simulink model "DDCU_wxt_v02_forA"  (R2014a)
settings: Solver=FixedStepDiscrete  StartTime=0.0  StopTime=50  FixedStep=0.0005  RelTol=1e-3
InitFcn:
  | Veh_Par_wxt
values from neighbouring files (symbols this model uses):
  ag_thr = 0.4*g    (= 3.924)    [Veh_Par_wxt.m]
  B = 2.25    [Veh_Par_wxt.m]
  bra_pre_em = 12    [Veh_Par_wxt.m]
  bra_pre_gz2 = 12/3    (= 4)    [Veh_Par_wxt.m]
  bra_pre_gz34 = 12/3    (= 4)    [Veh_Par_wxt.m]
  bra_pre_yd = 12/2    (= 6)    [Veh_Par_wxt.m]
  brakepre_dem_data = [0 1 2 3 4 5 6 7 8 9 10 11 12]    [Veh_Par_wxt.m]
  brakeTrq_dem_data = [0 218.198 436.396 654.594 872.792 1090.99 1309.188 1527.386 1745.584 1963.782 2181.98 2400.178 2618.376]    [Veh_Par_wxt.m]
  bratrq_max = 4*2618.376    (= 10473.504)    [Veh_Par_wxt.m]
  eff_tran = 0.75    [Veh_Par_wxt.m]
  G = Mass*g    (= 36297)    [Veh_Par_wxt.m]
  kd1 = 1    [Veh_Par_wxt.m]
  kd2 = 1    [Veh_Par_wxt.m]
  kd3 = 1    [Veh_Par_wxt.m]
  ki1 = 1    [Veh_Par_wxt.m]
  ki2 = 1    [Veh_Par_wxt.m]
  ki3 = 1    [Veh_Par_wxt.m]
  kp1 = 1    [Veh_Par_wxt.m]
  kp2 = 1    [Veh_Par_wxt.m]
  kp3 = 1    [Veh_Par_wxt.m]
  L = 3.12    [Veh_Par_wxt.m]
  Radius = 0.20    (= 0.2)    [Veh_Par_wxt.m]
  s_opt_yi_add = 0.05    [Veh_Par_wxt.m]
  s_opt_zhuan_add = 0.05    [Veh_Par_wxt.m]
  spd_map_mot = [0 100 200 300 360 400 500 600 700 800 900]*tras_ratio    [Veh_Par_wxt.m]
  speed_thr_park = 5/3.6/Radius*30/pi    (= 66.3145596216)    [Veh_Par_wxt.m]
  trq_map_mot = [1200 1200 1200 1200 1200 1080 864 720 617 540 480]/tras_ratio    [Veh_Par_wxt.m]
  v_thr1_b = 5    [Veh_Par_wxt.m]
  v_thr2_b = 20    [Veh_Par_wxt.m]
  v_thr_park = 5    [Veh_Par_wxt.m]
undefined symbols (not defined in the file or in its folder): DiscIntNeverNeededParam
libraries: simulink x201, ec5744lib x19
(part 9 of 9)

== matlab function DDCU_wxt_v02_forA/MainControl/mode_control/forward/forward/Brake/MATLAB Function5 ==
  data: bratrq_dem_lf input; bratrq_dem_lr input; bratrq_dem_rf input; bratrq_dem_rr input; flagyi_lf input; flagyi_lr input; bratrq_mot_lf output; flagyi_rf input; flagyi_rr input; bratrq_mot_lr output; bratrq_mot_rf output; bratrq_mot_rr output; bratrq_pid_lf input; bratrq_pid_lr input; bratrq_pid_rf input; bratrq_pid_rr input; brapre_out_l output; brapre_out_r output; gz_total input; v_act input; pwr_chg_bat input; trqlimL_dig_lf input; trqlimL_dig_lr input; trqlimL_dig_rf input; trqlimL_dig_rr input; speed_act_lf input; speed_act_lr input; speed_act_rf input; speed_act_rr input; v_thr1_b input; v_thr2_b input
function [bratrq_mot_lf,bratrq_mot_lr,bratrq_mot_rf,bratrq_mot_rr,brapre_out_l,brapre_out_r] = fcn(bratrq_dem_lf,bratrq_dem_lr,bratrq_dem_rf,bratrq_dem_rr,flagyi_lf,flagyi_lr,flagyi_rf,flagyi_rr,bratrq_pid_lf,bratrq_pid_lr,bratrq_pid_rf,bratrq_pid_rr,gz_total,v_act,pwr_chg_bat,trqlimL_dig_lf,trqlimL_dig_lr,trqlimL_dig_rf,trqlimL_dig_rr,speed_act_lf,speed_act_lr,speed_act_rf,speed_act_rr,v_thr1_b,v_thr2_b)
%#codegen pid模块在外面做，里面进行十六种情况的判断，先看一下效果，不能再修改。前轴单独控制，后轴低选控制
if flagyi_lf==0 && flagyi_lr==0 && flagyi_rf==0 && flagyi_rr==0 % 0电机滑移===============================================0电机滑移
    if gz_total==1  %电机有故障不进行制动能量回收，也不做ABS功能
        bratrq_mot_lf=0;
        bratrq_mot_lr=0;
        bratrq_mot_rf=0;
        bratrq_mot_rr=0;
        brapre_out_l=(bratrq_dem_lf+bratrq_dem_lr)/150;%除以150，对应Mpa
        brapre_out_r=(bratrq_dem_rf+bratrq_dem_rr)/150;
    else   %电机无故障，根据车速判断是否进行制动能量回收
        if   v_act<=v_thr1_b  %车速太小，机械制动
            bratrq_mot_lf=0;
            bratrq_mot_lr=0;
            bratrq_mot_rf=0;
            bratrq_mot_rr=0;
            brapre_out_l=(bratrq_dem_lf+bratrq_dem_lr)/150;%除以150，对应Mpa
            brapre_out_r=(bratrq_dem_rf+bratrq_dem_rr)/150;
        elseif v_act>v_thr1_b && v_act<=v_thr2_b %车速在5~20之间，复合制动
            bratrq_mot_lf1=bratrq_dem_lf*(v_act-v_thr1_b)/(v_thr2_b-v_thr1_b);
            bratrq_mot_lf2=9549*(pwr_chg_bat/4)/speed_act_lf;
            bratrq_mot_lf=min(trqlimL_dig_lf,min(bratrq_mot_lf1,bratrq_mot_lf2));
            
            bratrq_mot_lr1=bratrq_dem_lr*(v_act-v_thr1_b)/(v_thr2_b-v_thr1_b);
            bratrq_mot_lr2=9549*(pwr_chg_bat/4)/speed_act_lr;
            bratrq_mot_lr=min(trqlimL_dig_lr,min(bratrq_mot_lr1,bratrq_mot_lr2));
            
            bratrq_mot_rf1=bratrq_dem_rf*(v_act-v_thr1_b)/(v_thr2_b-v_thr1_b);
            bratrq_mot_rf2=9549*(pwr_chg_bat/4)/speed_act_rf;
            bratrq_mot_rf=min(trqlimL_dig_rf,min(bratrq_mot_rf1,bratrq_mot_rf2));
            
            bratrq_mot_rr1=bratrq_dem_rr*(v_act-v_thr1_b)/(v_thr2_b-v_thr1_b);
            bratrq_mot_rr2=9549*(pwr_chg_bat/4)/speed_act_rr;
            bratrq_mot_rr=min(trqlimL_dig_rr,min(bratrq_mot_rr1,bratrq_mot_rr2));
            
            brapre_out_l=((bratrq_dem_lf+bratrq_dem_lr)-(bratrq_mot_lf+bratrq_mot_lr))/150;
            brapre_out_r=((bratrq_dem_rf+bratrq_dem_rr)-(bratrq_mot_rf+bratrq_mot_rr))/150;
        else  %车速大于20，优先电制动
            bratrq_mot_lf1=bratrq_dem_lf;
            bratrq_mot_lf2=9549*(pwr_chg_bat/4)/speed_act_lf;
            bratrq_mot_lf=min(trqlimL_dig_lf,min(bratrq_mot_lf1,bratrq_mot_lf2));
            
            bratrq_mot_lr1=bratrq_dem_lr;
            bratrq_mot_lr2=9549*(pwr_chg_bat/4)/speed_act_lr;
            bratrq_mot_lr=min(trqlimL_dig_lr,min(bratrq_mot_lr1,bratrq_mot_lr2));
            
            bratrq_mot_rf1=bratrq_dem_rf;
            bratrq_mot_rf2=9549*(pwr_chg_bat/4)/speed_act_rf;
            bratrq_mot_rf=min(trqlimL_dig_rf,min(bratrq_mot_rf1,bratrq_mot_rf2));
            
            bratrq_mot_rr1=bratrq_dem_rr;
            bratrq_mot_rr2=9549*(pwr_chg_bat/4)/speed_act_rr;
            bratrq_mot_rr=min(trqlimL_dig_rr,min(bratrq_mot_rr1,bratrq_mot_rr2));
            
            brapre_out_l=((bratrq_dem_lf+bratrq_dem_lr)-(bratrq_mot_lf+bratrq_mot_lr))/150;
            brapre_out_r=((bratrq_dem_rf+bratrq_dem_rr)-(bratrq_mot_rf+bratrq_mot_rr))/150;
        end
    end
    
    
    
elseif flagyi_lf==1 && flagyi_lr==0 && flagyi_rf==0 && flagyi_rr==0 %左前轮滑移===================================================1电机滑移
    
    if gz_total==1  %电机有故障不进行制动能量回收，也不做ABS功能
        bratrq_mot_lf=0;
        bratrq_mot_lr=0;
        bratrq_mot_rf=0;
        bratrq_mot_rr=0;
        brapre_out_l=(bratrq_dem_lf+bratrq_dem_lr)/150;%除以150，对应Mpa
        brapre_out_r=(bratrq_dem_rf+bratrq_dem_rr)/150;
    else   %电机无故障，根据车速判断是否进行制动能量回收
        if   v_act<=v_thr1_b  %车速太小，机械制动
            bratrq_mot_lf=0;
            bratrq_mot_lr=0;
            bratrq_mot_rf=0;
            bratrq_mot_rr=0;
            brapre_out_l=(bratrq_dem_lf+bratrq_dem_lr)/150;%除以150，对应Mpa
            brapre_out_r=(bratrq_dem_rf+bratrq_dem_rr)/150;
        elseif v_act>v_thr1_b && v_act<=v_thr2_b %车速在5~20之间，复合制动
            bratrq_mot_lf1=bratrq_dem_lf*(v_act-v_thr1_b)/(v_thr2_b-v_thr1_b);
            bratrq_mot_lf2=9549*(pwr_chg_bat/4)/speed_act_lf;
            bratrq_mot_lf=min(trqlimL_dig_lf,min(bratrq_mot_lf1,bratrq_mot_lf2));
            
            bratrq_mot_lr1=bratrq_dem_lr*(v_act-v_thr1_b)/(v_thr2_b-v_thr1_b);
            bratrq_mot_lr2=9549*(pwr_chg_bat/4)/speed_act_lr;
            bratrq_mot_lr=min(trqlimL_dig_lr,min(bratrq_mot_lr1,bratrq_mot_lr2));
            
            bratrq_mot_rf1=bratrq_dem_rf*(v_act-v_thr1_b)/(v_thr2_b-v_thr1_b);
            bratrq_mot_rf2=9549*(pwr_chg_bat/4)/speed_act_rf;
            bratrq_mot_rf=min(trqlimL_dig_rf,min(bratrq_mot_rf1,bratrq_mot_rf2));
            
            bratrq_mot_rr1=bratrq_dem_rr*(v_act-v_thr1_b)/(v_thr2_b-v_thr1_b);
            bratrq_mot_rr2=9549*(pwr_chg_bat/4)/speed_act_rr;
            bratrq_mot_rr=min(trqlimL_dig_rr,min(bratrq_mot_rr1,bratrq_mot_rr2));
            
            brapre_out_l=((bratrq_dem_lf+bratrq_dem_lr)-(bratrq_mot_lf+bratrq_mot_lr))/150;
            brapre_out_r=((bratrq_dem_rf+bratrq_dem_rr)-(bratrq_mot_rf+bratrq_mot_rr))/150;
        else  %车速大于20，优先电制动,且进行ABS功能
            bratrq_mot_lf1=bratrq_dem_lf;
            bratrq_mot_lf2=9549*(pwr_chg_bat/4)/speed_act_lf;
            bratrq_mot_lf=min(trqlimL_dig_lf,min(bratrq_mot_lf1,bratrq_mot_lf2))+(bratrq_pid_lf-bratrq_dem_lf);
            
            bratrq_mot_lr1=bratrq_dem_lr;
            bratrq_mot_lr2=9549*(pwr_chg_bat/4)/speed_act_lr;
            bratrq_mot_lr=min(trqlimL_dig_lr,min(bratrq_mot_lr1,bratrq_mot_lr2));
            
            bratrq_mot_rf1=bratrq_dem_rf;
            bratrq_mot_rf2=9549*(pwr_chg_bat/4)/speed_act_rf;
            bratrq_mot_rf=min(trqlimL_dig_rf,min(bratrq_mot_rf1,bratrq_mot_rf2));
            
            bratrq_mot_rr1=bratrq_dem_rr;
            bratrq_mot_rr2=9549*(pwr_chg_bat/4)/speed_act_rr;
            bratrq_mot_rr=min(trqlimL_dig_rr,min(bratrq_mot_rr1,bratrq_mot_rr2));
            
            brapre_out_l=((bratrq_pid_lf+bratrq_dem_lr)-(bratrq_mot_lf+bratrq_mot_lr))/150;
            brapre_out_r=((bratrq_dem_rf+bratrq_dem_rr)-(bratrq_mot_rf+bratrq_mot_rr))/150;
        end
    end
    
    
elseif flagyi_lf==0 && flagyi_lr==1 && flagyi_rf==0 && flagyi_rr==0 %左后轮滑移,低选控制
    
    if gz_total==1  %电机有故障不进行制动能量回收，也不做ABS功能
        bratrq_mot_lf=0;
        bratrq_mot_lr=0;
        bratrq_mot_rf=0;
        bratrq_mot_rr=0;
        brapre_out_l=(bratrq_dem_lf+bratrq_dem_lr)/150;%除以150，对应Mpa
        brapre_out_r=(bratrq_dem_rf+bratrq_dem_rr)/150;
    else   %电机无故障，根据车速判断是否进行制动能量回收
        if   v_act<=v_thr1_b  %车速太小，机械制动
            bratrq_mot_lf=0;
            bratrq_mot_lr=0;
            bratrq_mot_rf=0;
            bratrq_mot_rr=0;
            brapre_out_l=(bratrq_dem_lf+bratrq_dem_lr)/150;%除以150，对应Mpa
            brapre_out_r=(bratrq_dem_rf+bratrq_dem_rr)/150;
        elseif v_act>v_thr1_b && v_act<=v_thr2_b %车速在5~20之间，复合制动
            bratrq_mot_lf1=bratrq_dem_lf*(v_act-v_thr1_b)/(v_thr2_b-v_thr1_b);
            bratrq_mot_lf2=9549*(pwr_chg_bat/4)/speed_act_lf;
            bratrq_mot_lf=min(trqlimL_dig_lf,min(bratrq_mot_lf1,bratrq_mot_lf2));
            
            bratrq_mot_lr1=bratrq_dem_lr*(v_act-v_thr1_b)/(v_thr2_b-v_thr1_b);
            bratrq_mot_lr2=9549*(pwr_chg_bat/4)/speed_act_lr;
            bratrq_mot_lr=min(trqlimL_dig_lr,min(bratrq_mot_lr1,bratrq_mot_lr2));
            
            bratrq_mot_rf1=bratrq_dem_rf*(v_act-v_thr1_b)/(v_thr2_b-v_thr1_b);
            bratrq_mot_rf2=9549*(pwr_chg_bat/4)/speed_act_rf;
            bratrq_mot_rf=min(trqlimL_dig_rf,min(bratrq_mot_rf1,bratrq_mot_rf2));
            
            bratrq_mot_rr1=bratrq_dem_rr*(v_act-v_thr1_b)/(v_thr2_b-v_thr1_b);
            bratrq_mot_rr2=9549*(pwr_chg_bat/4)/speed_act_rr;
            bratrq_mot_rr=min(trqlimL_dig_rr,min(bratrq_mot_rr1,bratrq_mot_rr2));
            
            brapre_out_l=((bratrq_dem_lf+bratrq_dem_lr)-(bratrq_mot_lf+bratrq_mot_lr))/150;
            brapre_out_r=((bratrq_dem_rf+bratrq_dem_rr)-(bratrq_mot_rf+bratrq_mot_rr))/150;
        else  %车速大于20，优先电制动,且进行ABS功能,左后降扭，右后同样得降扭啊。。。
            bratrq_mot_lf1=bratrq_dem_lf;
            bratrq_mot_lf2=9549*(pwr_chg_bat/4)/speed_act_lf;
            bratrq_mot_lf=min(trqlimL_dig_lf,min(bratrq_mot_lf1,bratrq_mot_lf2));
            
            bratrq_mot_lr1=bratrq_dem_lr;
            bratrq_mot_lr2=9549*(pwr_chg_bat/4)/speed_act_lr;
            bratrq_mot_lr=min(trqlimL_dig_lr,min(bratrq_mot_lr1,bratrq_mot_lr2))+(bratrq_pid_lr-bratrq_dem_lr);
            
            bratrq_mot_rf1=bratrq_dem_rf;
            bratrq_mot_rf2=9549*(pwr_chg_bat/4)/speed_act_rf;
            bratrq_mot_rf=min(trqlimL_dig_rf,min(bratrq_mot_rf1,bratrq_mot_rf2));
            
            bratrq_mot_rr1=bratrq_dem_rr;
            bratrq_mot_rr2=9549*(pwr_chg_bat/4)/speed_act_rr;
            bratrq_mot_rr=min(trqlimL_dig_rr,min(bratrq_mot_rr1,bratrq_mot_rr2))+(bratrq_pid_lr-bratrq_dem_lr);
            
            brapre_out_l=((bratrq_dem_lf+bratrq_pid_lr)-(bratrq_mot_lf+bratrq_mot_lr))/150;
            brapre_out_r=((bratrq_dem_rf+bratrq_dem_rr-(bratrq_pid_lr-bratrq_dem_lr))-(bratrq_mot_rf+bratrq_mot_rr))/150;
        end
    end
    
    
elseif flagyi_lf==0 && flagyi_lr==0 && flagyi_rf==1 && flagyi_rr==0 %右前轮滑移
    
    if gz_total==1  %电机有故障不进行制动能量回收，也不做ABS功能
        bratrq_mot_lf=0;
        bratrq_mot_lr=0;
        bratrq_mot_rf=0;
        bratrq_mot_rr=0;
        brapre_out_l=(bratrq_dem_lf+bratrq_dem_lr)/150;%除以150，对应Mpa
        brapre_out_r=(bratrq_dem_rf+bratrq_dem_rr)/150;
    else   %电机无故障，根据车速判断是否进行制动能量回收
        if   v_act<=v_thr1_b  %车速太小，机械制动
            bratrq_mot_lf=0;
            bratrq_mot_lr=0;
            bratrq_mot_rf=0;
            bratrq_mot_rr=0;
            brapre_out_l=(bratrq_dem_lf+bratrq_dem_lr)/150;%除以150，对应Mpa
            brapre_out_r=(bratrq_dem_rf+bratrq_dem_rr)/150;
        elseif v_act>v_thr1_b && v_act<=v_thr2_b %车速在5~20之间，复合制动
            bratrq_mot_lf1=bratrq_dem_lf*(v_act-v_thr1_b)/(v_thr2_b-v_thr1_b);
            bratrq_mot_lf2=9549*(pwr_chg_bat/4)/speed_act_lf;
            bratrq_mot_lf=min(trqlimL_dig_lf,min(bratrq_mot_lf1,bratrq_mot_lf2));
            
            bratrq_mot_lr1=bratrq_dem_lr*(v_act-v_thr1_b)/(v_thr2_b-v_thr1_b);
            bratrq_mot_lr2=9549*(pwr_chg_bat/4)/speed_act_lr;
            bratrq_mot_lr=min(trqlimL_dig_lr,min(bratrq_mot_lr1,bratrq_mot_lr2));
            
            bratrq_mot_rf1=bratrq_dem_rf*(v_act-v_thr1_b)/(v_thr2_b-v_thr1_b);
            bratrq_mot_rf2=9549*(pwr_chg_bat/4)/speed_act_rf;
            bratrq_mot_rf=min(trqlimL_dig_rf,min(bratrq_mot_rf1,bratrq_mot_rf2));
            
            bratrq_mot_rr1=bratrq_dem_rr*(v_act-v_thr1_b)/(v_thr2_b-v_thr1_b);
            bratrq_mot_rr2=9549*(pwr_chg_bat/4)/speed_act_rr;
            bratrq_mot_rr=min(trqlimL_dig_rr,min(bratrq_mot_rr1,bratrq_mot_rr2));
            
            brapre_out_l=((bratrq_dem_lf+bratrq_dem_lr)-(bratrq_mot_lf+bratrq_mot_lr))/150;
            brapre_out_r=((bratrq_dem_rf+bratrq_dem_rr)-(bratrq_mot_rf+bratrq_mot_rr))/150;
        else  %车速大于20，优先电制动,且进行ABS功能
            bratrq_mot_lf1=bratrq_dem_lf;
            bratrq_mot_lf2=9549*(pwr_chg_bat/4)/speed_act_lf;
            bratrq_mot_lf=min(trqlimL_dig_lf,min(bratrq_mot_lf1,bratrq_mot_lf2));
            
            bratrq_mot_lr1=bratrq_dem_lr;
            bratrq_mot_lr2=9549*(pwr_chg_bat/4)/speed_act_lr;
            bratrq_mot_lr=min(trqlimL_dig_lr,min(bratrq_mot_lr1,bratrq_mot_lr2));
            
            bratrq_mot_rf1=bratrq_dem_rf;
            bratrq_mot_rf2=9549*(pwr_chg_bat/4)/speed_act_rf;
            bratrq_mot_rf=min(trqlimL_dig_rf,min(bratrq_mot_rf1,bratrq_mot_rf2))+(bratrq_pid_rf-bratrq_dem_rf);
            
            bratrq_mot_rr1=bratrq_dem_rr;
            bratrq_mot_rr2=9549*(pwr_chg_bat/4)/speed_act_rr;
            bratrq_mot_rr=min(trqlimL_dig_rr,min(bratrq_mot_rr1,bratrq_mot_rr2));
            
            brapre_out_l=((bratrq_dem_lf+bratrq_dem_lr)-(bratrq_mot_lf+bratrq_mot_lr))/150;
            brapre_out_r=((bratrq_pid_rf+bratrq_dem_rr)-(bratrq_mot_rf+bratrq_mot_rr))/150;
        end
    end
    
    
elseif flagyi_lf==0 && flagyi_lr==0 && flagyi_rf==0 && flagyi_rr==1 %右后轮滑移
    
    if gz_total==1  %电机有故障不进行制动能量回收，也不做ABS功能
        bratrq_mot_lf=0;
        bratrq_mot_lr=0;
        bratrq_mot_rf=0;
        bratrq_mot_rr=0;
        brapre_out_l=(bratrq_dem_lf+bratrq_dem_lr)/150;%除以150，对应Mpa
        brapre_out_r=(bratrq_dem_rf+bratrq_dem_rr)/150;
    else   %电机无故障，根据车速判断是否进行制动能量回收
        if   v_act<=v_thr1_b  %车速太小，机械制动
            bratrq_mot_lf=0;
            bratrq_mot_lr=0;
            bratrq_mot_rf=0;
            bratrq_mot_rr=0;
            brapre_out_l=(bratrq_dem_lf+bratrq_dem_lr)/150;%除以150，对应Mpa
            brapre_out_r=(bratrq_dem_rf+bratrq_dem_rr)/150;
        elseif v_act>v_thr1_b && v_act<=v_thr2_b %车速在5~20之间，复合制动
            bratrq_mot_lf1=bratrq_dem_lf*(v_act-v_thr1_b)/(v_thr2_b-v_thr1_b);
            bratrq_mot_lf2=9549*(pwr_chg_bat/4)/speed_act_lf;
            bratrq_mot_lf=min(trqlimL_dig_lf,min(bratrq_mot_lf1,bratrq_mot_lf2));
            
            bratrq_mot_lr1=bratrq_dem_lr*(v_act-v_thr1_b)/(v_thr2_b-v_thr1_b);
            bratrq_mot_lr2=9549*(pwr_chg_bat/4)/speed_act_lr;
            bratrq_mot_lr=min(trqlimL_dig_lr,min(bratrq_mot_lr1,bratrq_mot_lr2));
            
            bratrq_mot_rf1=bratrq_dem_rf*(v_act-v_thr1_b)/(v_thr2_b-v_thr1_b);
            bratrq_mot_rf2=9549*(pwr_chg_bat/4)/speed_act_rf;
            bratrq_mot_rf=min(trqlimL_dig_rf,min(bratrq_mot_rf1,bratrq_mot_rf2));
            
            bratrq_mot_rr1=bratrq_dem_rr*(v_act-v_thr1_b)/(v_thr2_b-v_thr1_b);
            bratrq_mot_rr2=9549*(pwr_chg_bat/4)/speed_act_rr;
            bratrq_mot_rr=min(trqlimL_dig_rr,min(bratrq_mot_rr1,bratrq_mot_rr2));
            
            brapre_out_l=((bratrq_dem_lf+bratrq_dem_lr)-(bratrq_mot_lf+bratrq_mot_lr))/150;
            brapre_out_r=((bratrq_dem_rf+bratrq_dem_rr)-(bratrq_mot_rf+bratrq_mot_rr))/150;
        else  %车速大于20，优先电制动,且进行ABS功能,右后降扭，左后同样得降扭啊。。。
            
            bratrq_mot_rf1=bratrq_dem_rf;
            bratrq_mot_rf2=9549*(pwr_chg_bat/4)/speed_act_rf;
            bratrq_mot_rf=min(trqlimL_dig_rf,min(bratrq_mot_rf1,bratrq_mot_rf2));
            
            bratrq_mot_rr1=bratrq_dem_rr;
            bratrq_mot_rr2=9549*(pwr_chg_bat/4)/speed_act_rr;
            bratrq_mot_rr=min(trqlimL_dig_rr,min(bratrq_mot_rr1,bratrq_mot_rr2))+(bratrq_pid_rr-bratrq_dem_rr);
            
            bratrq_mot_lf1=bratrq_dem_lf;
            bratrq_mot_lf2=9549*(pwr_chg_bat/4)/speed_act_lf;
            bratrq_mot_lf=min(trqlimL_dig_lf,min(bratrq_mot_lf1,bratrq_mot_lf2));
            
            bratrq_mot_lr1=bratrq_dem_lr;
            bratrq_mot_lr2=9549*(pwr_chg_bat/4)/speed_act_lr;
            bratrq_mot_lr=min(trqlimL_dig_lr,min(bratrq_mot_lr1,bratrq_mot_lr2))+(bratrq_pid_rr-bratrq_dem_rr);
            
            
            
            brapre_out_l=((bratrq_dem_lf+bratrq_dem_lr-(bratrq_pid_rr-bratrq_dem_rr))-(bratrq_mot_lf+bratrq_mot_lr))/150;
            brapre_out_r=((bratrq_dem_rf+bratrq_pid_rr)-(bratrq_mot_rf+bratrq_mot_rr))/150;
        end
    end
    
    
elseif flagyi_lf==1 && flagyi_lr==1 && flagyi_rf==0 && flagyi_rr==0 %左侧两轮滑移=====================================================================2电机滑移
    
    if gz_total==1  %电机有故障不进行制动能量回收，也不做ABS功能
        bratrq_mot_lf=0;
        bratrq_mot_lr=0;
        bratrq_mot_rf=0;
        bratrq_mot_rr=0;
        brapre_out_l=(bratrq_dem_lf+bratrq_dem_lr)/150;%除以150，对应Mpa
        brapre_out_r=(bratrq_dem_rf+bratrq_dem_rr)/150;
    else   %电机无故障，根据车速判断是否进行制动能量回收
        if   v_act<=v_thr1_b  %车速太小，机械制动
            bratrq_mot_lf=0;
            bratrq_mot_lr=0;
            bratrq_mot_rf=0;
            bratrq_mot_rr=0;
            brapre_out_l=(bratrq_dem_lf+bratrq_dem_lr)/150;%除以150，对应Mpa
            brapre_out_r=(bratrq_dem_rf+bratrq_dem_rr)/150;
        elseif v_act>v_thr1_b && v_act<=v_thr2_b %车速在5~20之间，复合制动
            bratrq_mot_lf1=bratrq_dem_lf*(v_act-v_thr1_b)/(v_thr2_b-v_thr1_b);
            bratrq_mot_lf2=9549*(pwr_chg_bat/4)/speed_act_lf;
            bratrq_mot_lf=min(trqlimL_dig_lf,min(bratrq_mot_lf1,bratrq_mot_lf2));
            
            bratrq_mot_lr1=bratrq_dem_lr*(v_act-v_thr1_b)/(v_thr2_b-v_thr1_b);
            bratrq_mot_lr2=9549*(pwr_chg_bat/4)/speed_act_lr;
            bratrq_mot_lr=min(trqlimL_dig_lr,min(bratrq_mot_lr1,bratrq_mot_lr2));
            
            bratrq_mot_rf1=bratrq_dem_rf*(v_act-v_thr1_b)/(v_thr2_b-v_thr1_b);
            bratrq_mot_rf2=9549*(pwr_chg_bat/4)/speed_act_rf;
            bratrq_mot_rf=min(trqlimL_dig_rf,min(bratrq_mot_rf1,bratrq_mot_rf2));
            
            bratrq_mot_rr1=bratrq_dem_rr*(v_act-v_thr1_b)/(v_thr2_b-v_thr1_b);
            bratrq_mot_rr2=9549*(pwr_chg_bat/4)/speed_act_rr;
            bratrq_mot_rr=min(trqlimL_dig_rr,min(bratrq_mot_rr1,bratrq_mot_rr2));
            
            brapre_out_l=((bratrq_dem_lf+bratrq_dem_lr)-(bratrq_mot_lf+bratrq_mot_lr))/150;
            brapre_out_r=((bratrq_dem_rf+bratrq_dem_rr)-(bratrq_mot_rf+bratrq_mot_rr))/150;
        else  %车速大于20，优先电制动,且进行ABS功能
            bratrq_mot_lf1=bratrq_dem_lf;
            bratrq_mot_lf2=9549*(pwr_chg_bat/4)/speed_act_lf;
            bratrq_mot_lf=min(trqlimL_dig_lf,min(bratrq_mot_lf1,bratrq_mot_lf2))+(bratrq_pid_lf-bratrq_dem_lf);
            
            bratrq_mot_lr1=bratrq_dem_lr;
            bratrq_mot_lr2=9549*(pwr_chg_bat/4)/speed_act_lr;
            bratrq_mot_lr=min(trqlimL_dig_lr,min(bratrq_mot_lr1,bratrq_mot_lr2))+(bratrq_pid_lr-bratrq_dem_lr);
            
            bratrq_mot_rf1=bratrq_dem_rf;
            bratrq_mot_rf2=9549*(pwr_chg_bat/4)/speed_act_rf;
            bratrq_mot_rf=min(trqlimL_dig_rf,min(bratrq_mot_rf1,bratrq_mot_rf2));
            
            bratrq_mot_rr1=bratrq_dem_rr;
            bratrq_mot_rr2=9549*(pwr_chg_bat/4)/speed_act_rr;
            bratrq_mot_rr=min(trqlimL_dig_rr,min(bratrq_mot_rr1,bratrq_mot_rr2))+(bratrq_pid_lr-bratrq_dem_lr);
            
            brapre_out_l=((bratrq_pid_lf+bratrq_pid_lr)-(bratrq_mot_lf+bratrq_mot_lr))/150;
            brapre_out_r=((bratrq_dem_rf+bratrq_dem_rr-(bratrq_pid_lr-bratrq_dem_lr))-(bratrq_mot_rf+bratrq_mot_rr))/150;
        end
    end
    
    
elseif flagyi_lf==0 && flagyi_lr==0 && flagyi_rf==1 && flagyi_rr==1 %右侧两轮滑移
    
    if gz_total==1  %电机有故障不进行制动能量回收，也不做ABS功能
        bratrq_mot_lf=0;
        bratrq_mot_lr=0;
        bratrq_mot_rf=0;
        bratrq_mot_rr=0;
        brapre_out_l=(bratrq_dem_lf+bratrq_dem_lr)/150;%除以150，对应Mpa
        brapre_out_r=(bratrq_dem_rf+bratrq_dem_rr)/150;
    else   %电机无故障，根据车速判断是否进行制动能量回收
        if   v_act<=v_thr1_b  %车速太小，机械制动
            bratrq_mot_lf=0;
            bratrq_mot_lr=0;
            bratrq_mot_rf=0;
            bratrq_mot_rr=0;
            brapre_out_l=(bratrq_dem_lf+bratrq_dem_lr)/150;%除以150，对应Mpa
            brapre_out_r=(bratrq_dem_rf+bratrq_dem_rr)/150;
        elseif v_act>v_thr1_b && v_act<=v_thr2_b %车速在5~20之间，复合制动
            bratrq_mot_lf1=bratrq_dem_lf*(v_act-v_thr1_b)/(v_thr2_b-v_thr1_b);
            bratrq_mot_lf2=9549*(pwr_chg_bat/4)/speed_act_lf;
            bratrq_mot_lf=min(trqlimL_dig_lf,min(bratrq_mot_lf1,bratrq_mot_lf2));
            
            bratrq_mot_lr1=bratrq_dem_lr*(v_act-v_thr1_b)/(v_thr2_b-v_thr1_b);
            bratrq_mot_lr2=9549*(pwr_chg_bat/4)/speed_act_lr;
            bratrq_mot_lr=min(trqlimL_dig_lr,min(bratrq_mot_lr1,bratrq_mot_lr2));
            
            bratrq_mot_rf1=bratrq_dem_rf*(v_act-v_thr1_b)/(v_thr2_b-v_thr1_b);
            bratrq_mot_rf2=9549*(pwr_chg_bat/4)/speed_act_rf;
            bratrq_mot_rf=min(trqlimL_dig_rf,min(bratrq_mot_rf1,bratrq_mot_rf2));
            
            bratrq_mot_rr1=bratrq_dem_rr*(v_act-v_thr1_b)/(v_thr2_b-v_thr1_b);
            bratrq_mot_rr2=9549*(pwr_chg_bat/4)/speed_act_rr;
            bratrq_mot_rr=min(trqlimL_dig_rr,min(bratrq_mot_rr1,bratrq_mot_rr2));
            
            brapre_out_l=((bratrq_dem_lf+bratrq_dem_lr)-(bratrq_mot_lf+bratrq_mot_lr))/150;
            brapre_out_r=((bratrq_dem_rf+bratrq_dem_rr)-(bratrq_mot_rf+bratrq_mot_rr))/150;
        else  %车速大于20，优先电制动,且进行ABS功能
            bratrq_mot_rf1=bratrq_dem_rf;
            bratrq_mot_rf2=9549*(pwr_chg_bat/4)/speed_act_rf;
            bratrq_mot_rf=min(trqlimL_dig_rf,min(bratrq_mot_rf1,bratrq_mot_rf2))+(bratrq_pid_rf-bratrq_dem_rf);
            
            bratrq_mot_rr1=bratrq_dem_rr;
            bratrq_mot_rr2=9549*(pwr_chg_bat/4)/speed_act_rr;
            bratrq_mot_rr=min(trqlimL_dig_rr,min(bratrq_mot_rr1,bratrq_mot_rr2))+(bratrq_pid_rr-bratrq_dem_rr);
            
            bratrq_mot_lf1=bratrq_dem_lf;
            bratrq_mot_lf2=9549*(pwr_chg_bat/4)/speed_act_lf;
            bratrq_mot_lf=min(trqlimL_dig_lf,min(bratrq_mot_lf1,bratrq_mot_lf2));
            
            bratrq_mot_lr1=bratrq_dem_lr;
            bratrq_mot_lr2=9549*(pwr_chg_bat/4)/speed_act_lr;
            bratrq_mot_lr=min(trqlimL_dig_lr,min(bratrq_mot_lr1,bratrq_mot_lr2))+(bratrq_pid_rr-bratrq_dem_rr);
            
            
            
            brapre_out_l=((bratrq_pid_lf+bratrq_pid_lr-(bratrq_pid_rr-bratrq_dem_rr))-(bratrq_mot_lf+bratrq_mot_lr))/150;
            brapre_out_r=((bratrq_pid_rf+bratrq_pid_rr)-(bratrq_mot_rf+bratrq_mot_rr))/150;
        end
    end
    
    
elseif flagyi_lf==1 && flagyi_lr==0 && flagyi_rf==1 && flagyi_rr==0 %前轴滑移
    
    if gz_total==1  %电机有故障不进行制动能量回收，也不做ABS功能
        bratrq_mot_lf=0;
        bratrq_mot_lr=0;
        bratrq_mot_rf=0;
        bratrq_mot_rr=0;
        brapre_out_l=(bratrq_dem_lf+bratrq_dem_lr)/150;%除以150，对应Mpa
        brapre_out_r=(bratrq_dem_rf+bratrq_dem_rr)/150;
    else   %电机无故障，根据车速判断是否进行制动能量回收
        if   v_act<=v_thr1_b  %车速太小，机械制动
            bratrq_mot_lf=0;
            bratrq_mot_lr=0;
            bratrq_mot_rf=0;
            bratrq_mot_rr=0;
            brapre_out_l=(bratrq_dem_lf+bratrq_dem_lr)/150;%除以150，对应Mpa
            brapre_out_r=(bratrq_dem_rf+bratrq_dem_rr)/150;
        elseif v_act>v_thr1_b && v_act<=v_thr2_b %车速在5~20之间，复合制动
            bratrq_mot_lf1=bratrq_dem_lf*(v_act-v_thr1_b)/(v_thr2_b-v_thr1_b);
            bratrq_mot_lf2=9549*(pwr_chg_bat/4)/speed_act_lf;
            bratrq_mot_lf=min(trqlimL_dig_lf,min(bratrq_mot_lf1,bratrq_mot_lf2));
            
            bratrq_mot_lr1=bratrq_dem_lr*(v_act-v_thr1_b)/(v_thr2_b-v_thr1_b);
            bratrq_mot_lr2=9549*(pwr_chg_bat/4)/speed_act_lr;
            bratrq_mot_lr=min(trqlimL_dig_lr,min(bratrq_mot_lr1,bratrq_mot_lr2));
            
            bratrq_mot_rf1=bratrq_dem_rf*(v_act-v_thr1_b)/(v_thr2_b-v_thr1_b);
            bratrq_mot_rf2=9549*(pwr_chg_bat/4)/speed_act_rf;
            bratrq_mot_rf=min(trqlimL_dig_rf,min(bratrq_mot_rf1,bratrq_mot_rf2));
            
            bratrq_mot_rr1=bratrq_dem_rr*(v_act-v_thr1_b)/(v_thr2_b-v_thr1_b);
            bratrq_mot_rr2=9549*(pwr_chg_bat/4)/speed_act_rr;
            bratrq_mot_rr=min(trqlimL_dig_rr,min(bratrq_mot_rr1,bratrq_mot_rr2));
            
            brapre_out_l=((bratrq_dem_lf+bratrq_dem_lr)-(bratrq_mot_lf+bratrq_mot_lr))/150;
            brapre_out_r=((bratrq_dem_rf+bratrq_dem_rr)-(bratrq_mot_rf+bratrq_mot_rr))/150;
        else  %车速大于20，优先电制动,且进行ABS功能
            bratrq_mot_lf1=bratrq_dem_lf;
            bratrq_mot_lf2=9549*(pwr_chg_bat/4)/speed_act_lf;
            bratrq_mot_lf=min(trqlimL_dig_lf,min(bratrq_mot_lf1,bratrq_mot_lf2))+(bratrq_pid_lf-bratrq_dem_lf);
            
            bratrq_mot_lr1=bratrq_dem_lr;
            bratrq_mot_lr2=9549*(pwr_chg_bat/4)/speed_act_lr;
            bratrq_mot_lr=min(trqlimL_dig_lr,min(bratrq_mot_lr1,bratrq_mot_lr2));
            
            bratrq_mot_rf1=bratrq_dem_rf;
            bratrq_mot_rf2=9549*(pwr_chg_bat/4)/speed_act_rf;
            bratrq_mot_rf=min(trqlimL_dig_rf,min(bratrq_mot_rf1,bratrq_mot_rf2))+(bratrq_pid_rf-bratrq_dem_rf);
            
            bratrq_mot_rr1=bratrq_dem_rr;
            bratrq_mot_rr2=9549*(pwr_chg_bat/4)/speed_act_rr;
            bratrq_mot_rr=min(trqlimL_dig_rr,min(bratrq_mot_rr1,bratrq_mot_rr2));
            
            brapre_out_l=((bratrq_pid_lf+bratrq_dem_lr)-(bratrq_mot_lf+bratrq_mot_lr))/150;
            brapre_out_r=((bratrq_pid_rf+bratrq_dem_rr)-(bratrq_mot_rf+bratrq_mot_rr))/150;
        end
    end
    
    
elseif flagyi_lf==0 && flagyi_lr==1 && flagyi_rf==0 && flagyi_rr==1 %后轴滑移
    
    if gz_total==1  %电机有故障不进行制动能量回收，也不做ABS功能
        bratrq_mot_lf=0;
        bratrq_mot_lr=0;
        bratrq_mot_rf=0;
        bratrq_mot_rr=0;
        brapre_out_l=(bratrq_dem_lf+bratrq_dem_lr)/150;%除以150，对应Mpa
        brapre_out_r=(bratrq_dem_rf+bratrq_dem_rr)/150;
    else   %电机无故障，根据车速判断是否进行制动能量回收
        if   v_act<=v_thr1_b  %车速太小，机械制动
            bratrq_mot_lf=0;
            bratrq_mot_lr=0;
            bratrq_mot_rf=0;
            bratrq_mot_rr=0;
            brapre_out_l=(bratrq_dem_lf+bratrq_dem_lr)/150;%除以150，对应Mpa
            brapre_out_r=(bratrq_dem_rf+bratrq_dem_rr)/150;
        elseif v_act>v_thr1_b && v_act<=v_thr2_b %车速在5~20之间，复合制动
            bratrq_mot_lf1=bratrq_dem_lf*(v_act-v_thr1_b)/(v_thr2_b-v_thr1_b);
            bratrq_mot_lf2=9549*(pwr_chg_bat/4)/speed_act_lf;
            bratrq_mot_lf=min(trqlimL_dig_lf,min(bratrq_mot_lf1,bratrq_mot_lf2));
            
            bratrq_mot_lr1=bratrq_dem_lr*(v_act-v_thr1_b)/(v_thr2_b-v_thr1_b);
            bratrq_mot_lr2=9549*(pwr_chg_bat/4)/speed_act_lr;
            bratrq_mot_lr=min(trqlimL_dig_lr,min(bratrq_mot_lr1,bratrq_mot_lr2));
            
            bratrq_mot_rf1=bratrq_dem_rf*(v_act-v_thr1_b)/(v_thr2_b-v_thr1_b);
            bratrq_mot_rf2=9549*(pwr_chg_bat/4)/speed_act_rf;
            bratrq_mot_rf=min(trqlimL_dig_rf,min(bratrq_mot_rf1,bratrq_mot_rf2));
            
            bratrq_mot_rr1=bratrq_dem_rr*(v_act-v_thr1_b)/(v_thr2_b-v_thr1_b);
            bratrq_mot_rr2=9549*(pwr_chg_bat/4)/speed_act_rr;
            bratrq_mot_rr=min(trqlimL_dig_rr,min(bratrq_mot_rr1,bratrq_mot_rr2));
            
            brapre_out_l=((bratrq_dem_lf+bratrq_dem_lr)-(bratrq_mot_lf+bratrq_mot_lr))/150;
            brapre_out_r=((bratrq_dem_rf+bratrq_dem_rr)-(bratrq_mot_rf+bratrq_mot_rr))/150;
        else  %车速大于20，优先电制动,且进行ABS功能
            bratrq_mot_lf1=bratrq_dem_lf;
            bratrq_mot_lf2=9549*(pwr_chg_bat/4)/speed_act_lf;
            bratrq_mot_lf=min(trqlimL_dig_lf,min(bratrq_mot_lf1,bratrq_mot_lf2));
            
            bratrq_mot_rf1=bratrq_dem_rf;
            bratrq_mot_rf2=9549*(pwr_chg_bat/4)/speed_act_rf;
            bratrq_mot_rf=min(trqlimL_dig_rf,min(bratrq_mot_rf1,bratrq_mot_rf2));
            if (bratrq_pid_lr-bratrq_dem_lr)>(bratrq_pid_rr-bratrq_dem_rr)
                
                bratrq_mot_lr1=bratrq_dem_lr;
                bratrq_mot_lr2=9549*(pwr_chg_bat/4)/speed_act_lr;
                bratrq_mot_lr=min(trqlimL_dig_lr,min(bratrq_mot_lr1,bratrq_mot_lr2))+(bratrq_pid_rr-bratrq_dem_rr);
                
                
                
                bratrq_mot_rr1=bratrq_dem_rr;
                bratrq_mot_rr2=9549*(pwr_chg_bat/4)/speed_act_rr;
                bratrq_mot_rr=min(trqlimL_dig_rr,min(bratrq_mot_rr1,bratrq_mot_rr2))+(bratrq_pid_rr-bratrq_dem_rr);
                
                brapre_out_l=((bratrq_dem_lf+bratrq_dem_lr-(bratrq_pid_rr-bratrq_dem_rr))-(bratrq_mot_lf+bratrq_mot_lr))/150;
                brapre_out_r=((bratrq_dem_rf+bratrq_pid_rr)-(bratrq_mot_rf+bratrq_mot_rr))/150;
            else
                bratrq_mot_lr1=bratrq_dem_lr;
                bratrq_mot_lr2=9549*(pwr_chg_bat/4)/speed_act_lr;
                bratrq_mot_lr=min(trqlimL_dig_lr,min(bratrq_mot_lr1,bratrq_mot_lr2))+(bratrq_pid_lr-bratrq_dem_lr);
                
                
                
                bratrq_mot_rr1=bratrq_dem_rr;
                bratrq_mot_rr2=9549*(pwr_chg_bat/4)/speed_act_rr;
                bratrq_mot_rr=min(trqlimL_dig_rr,min(bratrq_mot_rr1,bratrq_mot_rr2))+(bratrq_pid_lr-bratrq_dem_lr);
                
                brapre_out_l=((bratrq_dem_lf+bratrq_pid_lr)-(bratrq_mot_lf+bratrq_mot_lr))/150;
                brapre_out_r=((bratrq_dem_rf+bratrq_dem_rr-(bratrq_pid_lr-bratrq_dem_lr))-(bratrq_mot_rf+bratrq_mot_rr))/150;
            end
        end
    end
    
    
elseif flagyi_lf==1 && flagyi_lr==0 && flagyi_rf==0 && flagyi_rr==1 %左前轮和右后轮滑移
    
    if gz_total==1  %电机有故障不进行制动能量回收，也不做ABS功能
        bratrq_mot_lf=0;
        bratrq_mot_lr=0;
        bratrq_mot_rf=0;
        bratrq_mot_rr=0;
        brapre_out_l=(bratrq_dem_lf+bratrq_dem_lr)/150;%除以150，对应Mpa
        brapre_out_r=(bratrq_dem_rf+bratrq_dem_rr)/150;
    else   %电机无故障，根据车速判断是否进行制动能量回收
        if   v_act<=v_thr1_b  %车速太小，机械制动
            bratrq_mot_lf=0;
            bratrq_mot_lr=0;
            bratrq_mot_rf=0;
            bratrq_mot_rr=0;
            brapre_out_l=(bratrq_dem_lf+bratrq_dem_lr)/150;%除以150，对应Mpa
            brapre_out_r=(bratrq_dem_rf+bratrq_dem_rr)/150;
        elseif v_act>v_thr1_b && v_act<=v_thr2_b %车速在5~20之间，复合制动
            bratrq_mot_lf1=bratrq_dem_lf*(v_act-v_thr1_b)/(v_thr2_b-v_thr1_b);
            bratrq_mot_lf2=9549*(pwr_chg_bat/4)/speed_act_lf;
            bratrq_mot_lf=min(trqlimL_dig_lf,min(bratrq_mot_lf1,bratrq_mot_lf2));
            
            bratrq_mot_lr1=bratrq_dem_lr*(v_act-v_thr1_b)/(v_thr2_b-v_thr1_b);
            bratrq_mot_lr2=9549*(pwr_chg_bat/4)/speed_act_lr;
            bratrq_mot_lr=min(trqlimL_dig_lr,min(bratrq_mot_lr1,bratrq_mot_lr2));
            
            bratrq_mot_rf1=bratrq_dem_rf*(v_act-v_thr1_b)/(v_thr2_b-v_thr1_b);
            bratrq_mot_rf2=9549*(pwr_chg_bat/4)/speed_act_rf;
            bratrq_mot_rf=min(trqlimL_dig_rf,min(bratrq_mot_rf1,bratrq_mot_rf2));
            
            bratrq_mot_rr1=bratrq_dem_rr*(v_act-v_thr1_b)/(v_thr2_b-v_thr1_b);
            bratrq_mot_rr2=9549*(pwr_chg_bat/4)/speed_act_rr;
            bratrq_mot_rr=min(trqlimL_dig_rr,min(bratrq_mot_rr1,bratrq_mot_rr2));
            
            brapre_out_l=((bratrq_dem_lf+bratrq_dem_lr)-(bratrq_mot_lf+bratrq_mot_lr))/150;
            brapre_out_r=((bratrq_dem_rf+bratrq_dem_rr)-(bratrq_mot_rf+bratrq_mot_rr))/150;
        else  %车速大于20，优先电制动,且进行ABS功能
            bratrq_mot_lf1=bratrq_dem_lf;
            bratrq_mot_lf2=9549*(pwr_chg_bat/4)/speed_act_lf;
            bratrq_mot_lf=min(trqlimL_dig_lf,min(bratrq_mot_lf1,bratrq_mot_lf2))+(bratrq_pid_lf-bratrq_dem_lf);
            
            bratrq_mot_rr1=bratrq_dem_rr;
            bratrq_mot_rr2=9549*(pwr_chg_bat/4)/speed_act_rr;
            bratrq_mot_rr=min(trqlimL_dig_rr,min(bratrq_mot_rr1,bratrq_mot_rr2))+(bratrq_pid_rr-bratrq_dem_rr);
            
            bratrq_mot_rf1=bratrq_dem_rf;
            bratrq_mot_rf2=9549*(pwr_chg_bat/4)/speed_act_rf;
            bratrq_mot_rf=min(trqlimL_dig_rf,min(bratrq_mot_rf1,bratrq_mot_rf2));
            
            bratrq_mot_lr1=bratrq_dem_lr;
            bratrq_mot_lr2=9549*(pwr_chg_bat/4)/speed_act_lr;
            bratrq_mot_lr=min(trqlimL_dig_lr,min(bratrq_mot_lr1,bratrq_mot_lr2))+(bratrq_pid_rr-bratrq_dem_rr);
            
            
            
            
            
            brapre_out_l=((bratrq_pid_lf+bratrq_dem_lr-(bratrq_pid_rr-bratrq_dem_rr))-(bratrq_mot_lf+bratrq_mot_lr))/150;
            brapre_out_r=((bratrq_dem_rf+bratrq_pid_rr)-(bratrq_mot_rf+bratrq_mot_rr))/150;
        end
    end
    
    
elseif flagyi_lf==0 && flagyi_lr==1 && flagyi_rf==1 && flagyi_rr==0 %左后轮和右前轮滑移
    
    if gz_total==1  %电机有故障不进行制动能量回收，也不做ABS功能
        bratrq_mot_lf=0;
        bratrq_mot_lr=0;
        bratrq_mot_rf=0;
        bratrq_mot_rr=0;
        brapre_out_l=(bratrq_dem_lf+bratrq_dem_lr)/150;%除以150，对应Mpa
        brapre_out_r=(bratrq_dem_rf+bratrq_dem_rr)/150;
    else   %电机无故障，根据车速判断是否进行制动能量回收
        if   v_act<=v_thr1_b  %车速太小，机械制动
            bratrq_mot_lf=0;
            bratrq_mot_lr=0;
            bratrq_mot_rf=0;
            bratrq_mot_rr=0;
            brapre_out_l=(bratrq_dem_lf+bratrq_dem_lr)/150;%除以150，对应Mpa
            brapre_out_r=(bratrq_dem_rf+bratrq_dem_rr)/150;
        elseif v_act>v_thr1_b && v_act<=v_thr2_b %车速在5~20之间，复合制动
            bratrq_mot_lf1=bratrq_dem_lf*(v_act-v_thr1_b)/(v_thr2_b-v_thr1_b);
            bratrq_mot_lf2=9549*(pwr_chg_bat/4)/speed_act_lf;
            bratrq_mot_lf=min(trqlimL_dig_lf,min(bratrq_mot_lf1,bratrq_mot_lf2));
            
            bratrq_mot_lr1=bratrq_dem_lr*(v_act-v_thr1_b)/(v_thr2_b-v_thr1_b);
            bratrq_mot_lr2=9549*(pwr_chg_bat/4)/speed_act_lr;
            bratrq_mot_lr=min(trqlimL_dig_lr,min(bratrq_mot_lr1,bratrq_mot_lr2));
            
            bratrq_mot_rf1=bratrq_dem_rf*(v_act-v_thr1_b)/(v_thr2_b-v_thr1_b);
            bratrq_mot_rf2=9549*(pwr_chg_bat/4)/speed_act_rf;
            bratrq_mot_rf=min(trqlimL_dig_rf,min(bratrq_mot_rf1,bratrq_mot_rf2));
            
            bratrq_mot_rr1=bratrq_dem_rr*(v_act-v_thr1_b)/(v_thr2_b-v_thr1_b);
            bratrq_mot_rr2=9549*(pwr_chg_bat/4)/speed_act_rr;
            bratrq_mot_rr=min(trqlimL_dig_rr,min(bratrq_mot_rr1,bratrq_mot_rr2));
            
            brapre_out_l=((bratrq_dem_lf+bratrq_dem_lr)-(bratrq_mot_lf+bratrq_mot_lr))/150;
            brapre_out_r=((bratrq_dem_rf+bratrq_dem_rr)-(bratrq_mot_rf+bratrq_mot_rr))/150;
        else  %车速大于20，优先电制动,且进行ABS功能
            
            bratrq_mot_rf1=bratrq_dem_rf;
            bratrq_mot_rf2=9549*(pwr_chg_bat/4)/speed_act_rf;
            bratrq_mot_rf=min(trqlimL_dig_rf,min(bratrq_mot_rf1,bratrq_mot_rf2))+(bratrq_pid_rf-bratrq_dem_rf);
            
            bratrq_mot_lr1=bratrq_dem_lr;
            bratrq_mot_lr2=9549*(pwr_chg_bat/4)/speed_act_lr;
            bratrq_mot_lr=min(trqlimL_dig_lr,min(bratrq_mot_lr1,bratrq_mot_lr2))+(bratrq_pid_lf-bratrq_dem_lf);
            
            bratrq_mot_lf1=bratrq_dem_lf;
            bratrq_mot_lf2=9549*(pwr_chg_bat/4)/speed_act_lf;
            bratrq_mot_lf=min(trqlimL_dig_lf,min(bratrq_mot_lf1,bratrq_mot_lf2));
            
            bratrq_mot_rr1=bratrq_dem_rr;
            bratrq_mot_rr2=9549*(pwr_chg_bat/4)/speed_act_rr;
            bratrq_mot_rr=min(trqlimL_dig_rr,min(bratrq_mot_rr1,bratrq_mot_rr2))+(bratrq_pid_lr-bratrq_dem_lr);
            
            brapre_out_l=((bratrq_dem_lf+bratrq_pid_lr)-(bratrq_mot_lf+bratrq_mot_lr))/150;
            brapre_out_r=((bratrq_pid_rf+bratrq_dem_rr-(bratrq_pid_lr-bratrq_dem_lr))-(bratrq_mot_rf+bratrq_mot_rr))/150;
        end
    end
    
    
elseif flagyi_lf==1 && flagyi_lr==1 && flagyi_rf==1 && flagyi_rr==0 %右后不滑移======================================================================3电机滑移
    
    if gz_total==1  %电机有故障不进行制动能量回收，也不做ABS功能
        bratrq_mot_lf=0;
        bratrq_mot_lr=0;
        bratrq_mot_rf=0;
        bratrq_mot_rr=0;
        brapre_out_l=(bratrq_dem_lf+bratrq_dem_lr)/150;%除以150，对应Mpa
        brapre_out_r=(bratrq_dem_rf+bratrq_dem_rr)/150;
    else   %电机无故障，根据车速判断是否进行制动能量回收
        if   v_act<=v_thr1_b  %车速太小，机械制动
            bratrq_mot_lf=0;
            bratrq_mot_lr=0;
            bratrq_mot_rf=0;
            bratrq_mot_rr=0;
            brapre_out_l=(bratrq_dem_lf+bratrq_dem_lr)/150;%除以150，对应Mpa
            brapre_out_r=(bratrq_dem_rf+bratrq_dem_rr)/150;
        elseif v_act>v_thr1_b && v_act<=v_thr2_b %车速在5~20之间，复合制动
            bratrq_mot_lf1=bratrq_dem_lf*(v_act-v_thr1_b)/(v_thr2_b-v_thr1_b);
            bratrq_mot_lf2=9549*(pwr_chg_bat/4)/speed_act_lf;
            bratrq_mot_lf=min(trqlimL_dig_lf,min(bratrq_mot_lf1,bratrq_mot_lf2));
            
            bratrq_mot_lr1=bratrq_dem_lr*(v_act-v_thr1_b)/(v_thr2_b-v_thr1_b);
            bratrq_mot_lr2=9549*(pwr_chg_bat/4)/speed_act_lr;
            bratrq_mot_lr=min(trqlimL_dig_lr,min(bratrq_mot_lr1,bratrq_mot_lr2));
            
            bratrq_mot_rf1=bratrq_dem_rf*(v_act-v_thr1_b)/(v_thr2_b-v_thr1_b);
            bratrq_mot_rf2=9549*(pwr_chg_bat/4)/speed_act_rf;
            bratrq_mot_rf=min(trqlimL_dig_rf,min(bratrq_mot_rf1,bratrq_mot_rf2));
            
            bratrq_mot_rr1=bratrq_dem_rr*(v_act-v_thr1_b)/(v_thr2_b-v_thr1_b);
            bratrq_mot_rr2=9549*(pwr_chg_bat/4)/speed_act_rr;
            bratrq_mot_rr=min(trqlimL_dig_rr,min(bratrq_mot_rr1,bratrq_mot_rr2));
            
            brapre_out_l=((bratrq_dem_lf+bratrq_dem_lr)-(bratrq_mot_lf+bratrq_mot_lr))/150;
            brapre_out_r=((bratrq_dem_rf+bratrq_dem_rr)-(bratrq_mot_rf+bratrq_mot_rr))/150;
        else  %车速大于20，优先电制动,且进行ABS功能
            bratrq_mot_lf1=bratrq_dem_lf;
            bratrq_mot_lf2=9549*(pwr_chg_bat/4)/speed_act_lf;
            bratrq_mot_lf=min(trqlimL_dig_lf,min(bratrq_mot_lf1,bratrq_mot_lf2))+(bratrq_pid_lf-bratrq_dem_lf);
            
            bratrq_mot_lr1=bratrq_dem_lr;
            bratrq_mot_lr2=9549*(pwr_chg_bat/4)/speed_act_lr;
            bratrq_mot_lr=min(trqlimL_dig_lr,min(bratrq_mot_lr1,bratrq_mot_lr2))+(bratrq_pid_lr-bratrq_dem_lr);
            
            bratrq_mot_rf1=bratrq_dem_rf;
            bratrq_mot_rf2=9549*(pwr_chg_bat/4)/speed_act_rf;
            bratrq_mot_rf=min(trqlimL_dig_rf,min(bratrq_mot_rf1,bratrq_mot_rf2))+(bratrq_pid_rf-bratrq_dem_rf);
            
            bratrq_mot_rr1=bratrq_dem_rr;
            bratrq_mot_rr2=9549*(pwr_chg_bat/4)/speed_act_rr;
            bratrq_mot_rr=min(trqlimL_dig_rr,min(bratrq_mot_rr1,bratrq_mot_rr2))+(bratrq_pid_lr-bratrq_dem_lr);
            
            brapre_out_l=((bratrq_pid_lf+bratrq_pid_lr)-(bratrq_mot_lf+bratrq_mot_lr))/150;
            brapre_out_r=((bratrq_pid_rf+bratrq_dem_rr-(bratrq_pid_lr-bratrq_dem_lr))-(bratrq_mot_rf+bratrq_mot_rr))/150;
        end
    end
    
    
elseif flagyi_lf==1 && flagyi_lr==1 && flagyi_rf==0 && flagyi_rr==1 %右前不滑移
    
    if gz_total==1  %电机有故障不进行制动能量回收，也不做ABS功能
        bratrq_mot_lf=0;
        bratrq_mot_lr=0;
        bratrq_mot_rf=0;
        bratrq_mot_rr=0;
        brapre_out_l=(bratrq_dem_lf+bratrq_dem_lr)/150;%除以150，对应Mpa
        brapre_out_r=(bratrq_dem_rf+bratrq_dem_rr)/150;
    else   %电机无故障，根据车速判断是否进行制动能量回收
        if   v_act<=v_thr1_b  %车速太小，机械制动
            bratrq_mot_lf=0;
            bratrq_mot_lr=0;
            bratrq_mot_rf=0;
            bratrq_mot_rr=0;
            brapre_out_l=(bratrq_dem_lf+bratrq_dem_lr)/150;%除以150，对应Mpa
            brapre_out_r=(bratrq_dem_rf+bratrq_dem_rr)/150;
        elseif v_act>v_thr1_b && v_act<=v_thr2_b %车速在5~20之间，复合制动
            bratrq_mot_lf1=bratrq_dem_lf*(v_act-v_thr1_b)/(v_thr2_b-v_thr1_b);
            bratrq_mot_lf2=9549*(pwr_chg_bat/4)/speed_act_lf;
            bratrq_mot_lf=min(trqlimL_dig_lf,min(bratrq_mot_lf1,bratrq_mot_lf2));
            
            bratrq_mot_lr1=bratrq_dem_lr*(v_act-v_thr1_b)/(v_thr2_b-v_thr1_b);
            bratrq_mot_lr2=9549*(pwr_chg_bat/4)/speed_act_lr;
            bratrq_mot_lr=min(trqlimL_dig_lr,min(bratrq_mot_lr1,bratrq_mot_lr2));
            
            bratrq_mot_rf1=bratrq_dem_rf*(v_act-v_thr1_b)/(v_thr2_b-v_thr1_b);
            bratrq_mot_rf2=9549*(pwr_chg_bat/4)/speed_act_rf;
            bratrq_mot_rf=min(trqlimL_dig_rf,min(bratrq_mot_rf1,bratrq_mot_rf2));
            
            bratrq_mot_rr1=bratrq_dem_rr*(v_act-v_thr1_b)/(v_thr2_b-v_thr1_b);
            bratrq_mot_rr2=9549*(pwr_chg_bat/4)/speed_act_rr;
            bratrq_mot_rr=min(trqlimL_dig_rr,min(bratrq_mot_rr1,bratrq_mot_rr2));
            
            brapre_out_l=((bratrq_dem_lf+bratrq_dem_lr)-(bratrq_mot_lf+bratrq_mot_lr))/150;
            brapre_out_r=((bratrq_dem_rf+bratrq_dem_rr)-(bratrq_mot_rf+bratrq_mot_rr))/150;
        else  %车速大于20，优先电制动,且进行ABS功能
            bratrq_mot_lf1=bratrq_dem_lf;
            bratrq_mot_lf2=9549*(pwr_chg_bat/4)/speed_act_lf;
            bratrq_mot_lf=min(trqlimL_dig_lf,min(bratrq_mot_lf1,bratrq_mot_lf2))+(bratrq_pid_lf-bratrq_dem_lf);
            
            bratrq_mot_rf1=bratrq_dem_rf;
            bratrq_mot_rf2=9549*(pwr_chg_bat/4)/speed_act_rf;
            bratrq_mot_rf=min(trqlimL_dig_rf,min(bratrq_mot_rf1,bratrq_mot_rf2));
            
            if (bratrq_pid_lr-bratrq_dem_lr)>(bratrq_pid_rr-bratrq_dem_rr)
                
                bratrq_mot_lr1=bratrq_dem_lr;
                bratrq_mot_lr2=9549*(pwr_chg_bat/4)/speed_act_lr;
                bratrq_mot_lr=min(trqlimL_dig_lr,min(bratrq_mot_lr1,bratrq_mot_lr2))+(bratrq_pid_rr-bratrq_dem_rr);
                
                
                
                bratrq_mot_rr1=bratrq_dem_rr;
                bratrq_mot_rr2=9549*(pwr_chg_bat/4)/speed_act_rr;
                bratrq_mot_rr=min(trqlimL_dig_rr,min(bratrq_mot_rr1,bratrq_mot_rr2))+(bratrq_pid_rr-bratrq_dem_rr);
                
                brapre_out_l=((bratrq_pid_lf+bratrq_dem_lr-(bratrq_pid_rr-bratrq_dem_rr))-(bratrq_mot_lf+bratrq_mot_lr))/150;
                brapre_out_r=((bratrq_dem_rf+bratrq_pid_rr)-(bratrq_mot_rf+bratrq_mot_rr))/150;
                
            else
                bratrq_mot_lr1=bratrq_dem_lr;
                bratrq_mot_lr2=9549*(pwr_chg_bat/4)/speed_act_lr;
                bratrq_mot_lr=min(trqlimL_dig_lr,min(bratrq_mot_lr1,bratrq_mot_lr2))+(bratrq_pid_lr-bratrq_dem_lr);
                
                
                
                bratrq_mot_rr1=bratrq_dem_rr;
                bratrq_mot_rr2=9549*(pwr_chg_bat/4)/speed_act_rr;
                bratrq_mot_rr=min(trqlimL_dig_rr,min(bratrq_mot_rr1,bratrq_mot_rr2))+(bratrq_pid_lr-bratrq_dem_lr);
                
                brapre_out_l=((bratrq_pid_lf+bratrq_pid_lr)-(bratrq_mot_lf+bratrq_mot_lr))/150;
                brapre_out_r=((bratrq_dem_rf+bratrq_dem_rr-(bratrq_pid_lr-bratrq_dem_lr))-(bratrq_mot_rf+bratrq_mot_rr))/150;
            end
        end
    end
    
    
elseif flagyi_lf==1 && flagyi_lr==0 && flagyi_rf==1 && flagyi_rr==1 %左后不滑移
    
    if gz_total==1  %电机有故障不进行制动能量回收，也不做ABS功能
        bratrq_mot_lf=0;
        bratrq_mot_lr=0;
        bratrq_mot_rf=0;
        bratrq_mot_rr=0;
        brapre_out_l=(bratrq_dem_lf+bratrq_dem_lr)/150;%除以150，对应Mpa
        brapre_out_r=(bratrq_dem_rf+bratrq_dem_rr)/150;
    else   %电机无故障，根据车速判断是否进行制动能量回收
        if   v_act<=v_thr1_b  %车速太小，机械制动
            bratrq_mot_lf=0;
            bratrq_mot_lr=0;
            bratrq_mot_rf=0;
            bratrq_mot_rr=0;
            brapre_out_l=(bratrq_dem_lf+bratrq_dem_lr)/150;%除以150，对应Mpa
            brapre_out_r=(bratrq_dem_rf+bratrq_dem_rr)/150;
        elseif v_act>v_thr1_b && v_act<=v_thr2_b %车速在5~20之间，复合制动
            bratrq_mot_lf1=bratrq_dem_lf*(v_act-v_thr1_b)/(v_thr2_b-v_thr1_b);
            bratrq_mot_lf2=9549*(pwr_chg_bat/4)/speed_act_lf;
            bratrq_mot_lf=min(trqlimL_dig_lf,min(bratrq_mot_lf1,bratrq_mot_lf2));
            
            bratrq_mot_lr1=bratrq_dem_lr*(v_act-v_thr1_b)/(v_thr2_b-v_thr1_b);
            bratrq_mot_lr2=9549*(pwr_chg_bat/4)/speed_act_lr;
            bratrq_mot_lr=min(trqlimL_dig_lr,min(bratrq_mot_lr1,bratrq_mot_lr2));
            
            bratrq_mot_rf1=bratrq_dem_rf*(v_act-v_thr1_b)/(v_thr2_b-v_thr1_b);
            bratrq_mot_rf2=9549*(pwr_chg_bat/4)/speed_act_rf;
            bratrq_mot_rf=min(trqlimL_dig_rf,min(bratrq_mot_rf1,bratrq_mot_rf2));
            
            bratrq_mot_rr1=bratrq_dem_rr*(v_act-v_thr1_b)/(v_thr2_b-v_thr1_b);
            bratrq_mot_rr2=9549*(pwr_chg_bat/4)/speed_act_rr;
            bratrq_mot_rr=min(trqlimL_dig_rr,min(bratrq_mot_rr1,bratrq_mot_rr2));
            
            brapre_out_l=((bratrq_dem_lf+bratrq_dem_lr)-(bratrq_mot_lf+bratrq_mot_lr))/150;
            brapre_out_r=((bratrq_dem_rf+bratrq_dem_rr)-(bratrq_mot_rf+bratrq_mot_rr))/150;
        else  %车速大于20，优先电制动,且进行ABS功能
            bratrq_mot_lf1=bratrq_dem_lf;
            bratrq_mot_lf2=9549*(pwr_chg_bat/4)/speed_act_lf;
            bratrq_mot_lf=min(trqlimL_dig_lf,min(bratrq_mot_lf1,bratrq_mot_lf2))+(bratrq_pid_lf-bratrq_dem_lf);
            
            bratrq_mot_rf1=bratrq_dem_rf;
            bratrq_mot_rf2=9549*(pwr_chg_bat/4)/speed_act_rf;
            bratrq_mot_rf=min(trqlimL_dig_rf,min(bratrq_mot_rf1,bratrq_mot_rf2))+(bratrq_pid_rf-bratrq_dem_rf);
            
            
            bratrq_mot_rr1=bratrq_dem_rr;
            bratrq_mot_rr2=9549*(pwr_chg_bat/4)/speed_act_rr;
            bratrq_mot_rr=min(trqlimL_dig_rr,min(bratrq_mot_rr1,bratrq_mot_rr2))+(bratrq_pid_rr-bratrq_dem_rr);
            
            bratrq_mot_lr1=bratrq_dem_lr;
            bratrq_mot_lr2=9549*(pwr_chg_bat/4)/speed_act_lr;
            bratrq_mot_lr=min(trqlimL_dig_lr,min(bratrq_mot_lr1,bratrq_mot_lr2))+(bratrq_pid_rr-bratrq_dem_rr);
            
            
            
            
            brapre_out_l=((bratrq_pid_lf+bratrq_dem_lr-(bratrq_pid_rr-bratrq_dem_rr))-(bratrq_mot_lf+bratrq_mot_lr))/150;
            brapre_out_r=((bratrq_pid_rf+bratrq_pid_rr)-(bratrq_mot_rf+bratrq_mot_rr))/150;
        end
    end
    
    
elseif flagyi_lf==0 && flagyi_lr==1 && flagyi_rf==1 && flagyi_rr==1 %左前不滑移
    
    if gz_total==1  %电机有故障不进行制动能量回收，也不做ABS功能
        bratrq_mot_lf=0;
        bratrq_mot_lr=0;
        bratrq_mot_rf=0;
        bratrq_mot_rr=0;
        brapre_out_l=(bratrq_dem_lf+bratrq_dem_lr)/150;%除以150，对应Mpa
        brapre_out_r=(bratrq_dem_rf+bratrq_dem_rr)/150;
    else   %电机无故障，根据车速判断是否进行制动能量回收
        if   v_act<=v_thr1_b  %车速太小，机械制动
            bratrq_mot_lf=0;
            bratrq_mot_lr=0;
            bratrq_mot_rf=0;
            bratrq_mot_rr=0;
            brapre_out_l=(bratrq_dem_lf+bratrq_dem_lr)/150;%除以150，对应Mpa
            brapre_out_r=(bratrq_dem_rf+bratrq_dem_rr)/150;
        elseif v_act>v_thr1_b && v_act<=v_thr2_b %车速在5~20之间，复合制动
            bratrq_mot_lf1=bratrq_dem_lf*(v_act-v_thr1_b)/(v_thr2_b-v_thr1_b);
            bratrq_mot_lf2=9549*(pwr_chg_bat/4)/speed_act_lf;
            bratrq_mot_lf=min(trqlimL_dig_lf,min(bratrq_mot_lf1,bratrq_mot_lf2));
            
            bratrq_mot_lr1=bratrq_dem_lr*(v_act-v_thr1_b)/(v_thr2_b-v_thr1_b);
            bratrq_mot_lr2=9549*(pwr_chg_bat/4)/speed_act_lr;
            bratrq_mot_lr=min(trqlimL_dig_lr,min(bratrq_mot_lr1,bratrq_mot_lr2));
            
            bratrq_mot_rf1=bratrq_dem_rf*(v_act-v_thr1_b)/(v_thr2_b-v_thr1_b);
            bratrq_mot_rf2=9549*(pwr_chg_bat/4)/speed_act_rf;
            bratrq_mot_rf=min(trqlimL_dig_rf,min(bratrq_mot_rf1,bratrq_mot_rf2));
            
            bratrq_mot_rr1=bratrq_dem_rr*(v_act-v_thr1_b)/(v_thr2_b-v_thr1_b);
            bratrq_mot_rr2=9549*(pwr_chg_bat/4)/speed_act_rr;
            bratrq_mot_rr=min(trqlimL_dig_rr,min(bratrq_mot_rr1,bratrq_mot_rr2));
            
            brapre_out_l=((bratrq_dem_lf+bratrq_dem_lr)-(bratrq_mot_lf+bratrq_mot_lr))/150;
            brapre_out_r=((bratrq_dem_rf+bratrq_dem_rr)-(bratrq_mot_rf+bratrq_mot_rr))/150;
        else  %车速大于20，优先电制动,且进行ABS功能
            bratrq_mot_lf1=bratrq_dem_lf;
            bratrq_mot_lf2=9549*(pwr_chg_bat/4)/speed_act_lf;
            bratrq_mot_lf=min(trqlimL_dig_lf,min(bratrq_mot_lf1,bratrq_mot_lf2));
            
            bratrq_mot_rf1=bratrq_dem_rf;
            bratrq_mot_rf2=9549*(pwr_chg_bat/4)/speed_act_rf;
            bratrq_mot_rf=min(trqlimL_dig_rf,min(bratrq_mot_rf1,bratrq_mot_rf2))+(bratrq_pid_rf-bratrq_dem_rf);
            if (bratrq_pid_lr-bratrq_dem_lr)>(bratrq_pid_rr-bratrq_dem_rr)
                
                bratrq_mot_lr1=bratrq_dem_lr;
                bratrq_mot_lr2=9549*(pwr_chg_bat/4)/speed_act_lr;
                bratrq_mot_lr=min(trqlimL_dig_lr,min(bratrq_mot_lr1,bratrq_mot_lr2))+(bratrq_pid_rr-bratrq_dem_rr);
                
                
                
                bratrq_mot_rr1=bratrq_dem_rr;
                bratrq_mot_rr2=9549*(pwr_chg_bat/4)/speed_act_rr;
                bratrq_mot_rr=min(trqlimL_dig_rr,min(bratrq_mot_rr1,bratrq_mot_rr2))+(bratrq_pid_rr-bratrq_dem_rr);
                
                brapre_out_l=((bratrq_dem_lf+bratrq_dem_lr-(bratrq_pid_rr-bratrq_dem_rr))-(bratrq_mot_lf+bratrq_mot_lr))/150;
                brapre_out_r=((bratrq_pid_rf+bratrq_pid_rr)-(bratrq_mot_rf+bratrq_mot_rr))/150;
            else
                bratrq_mot_lr1=bratrq_dem_lr;
                bratrq_mot_lr2=9549*(pwr_chg_bat/4)/speed_act_lr;
                bratrq_mot_lr=min(trqlimL_dig_lr,min(bratrq_mot_lr1,bratrq_mot_lr2))+(bratrq_pid_lr-bratrq_dem_lr);
                
                
                
                bratrq_mot_rr1=bratrq_dem_rr;
                bratrq_mot_rr2=9549*(pwr_chg_bat/4)/speed_act_rr;
                bratrq_mot_rr=min(trqlimL_dig_rr,min(bratrq_mot_rr1,bratrq_mot_rr2))+(bratrq_pid_lr-bratrq_dem_lr);
                
                brapre_out_l=((bratrq_dem_lf+bratrq_pid_lr)-(bratrq_mot_lf+bratrq_mot_lr))/150;
                brapre_out_r=((bratrq_pid_rf+bratrq_dem_rr-(bratrq_pid_lr-bratrq_dem_lr))-(bratrq_mot_rf+bratrq_mot_rr))/150;
            end
        end
    end
    
    
else
    %     flagyi_lf==1 && flagyi_lr==1 && flagyi_rf==1 && flagyi_rr==1 %4电机均滑移======================================================================4电机均滑移
    
    if gz_total==1  %电机有故障不进行制动能量回收，也不做ABS功能
        bratrq_mot_lf=0;
        bratrq_mot_lr=0;
        bratrq_mot_rf=0;
        bratrq_mot_rr=0;
        brapre_out_l=(bratrq_dem_lf+bratrq_dem_lr)/150;%除以150，对应Mpa
        brapre_out_r=(bratrq_dem_rf+bratrq_dem_rr)/150;
    else   %电机无故障，根据车速判断是否进行制动能量回收
        if   v_act<=v_thr1_b  %车速太小，机械制动
            bratrq_mot_lf=0;
            bratrq_mot_lr=0;
            bratrq_mot_rf=0;
            bratrq_mot_rr=0;
            brapre_out_l=(bratrq_dem_lf+bratrq_dem_lr)/150;%除以150，对应Mpa
            brapre_out_r=(bratrq_dem_rf+bratrq_dem_rr)/150;
        elseif v_act>v_thr1_b && v_act<=v_thr2_b %车速在5~20之间，复合制动
            bratrq_mot_lf1=bratrq_dem_lf*(v_act-v_thr1_b)/(v_thr2_b-v_thr1_b);
            bratrq_mot_lf2=9549*(pwr_chg_bat/4)/speed_act_lf;
            bratrq_mot_lf=min(trqlimL_dig_lf,min(bratrq_mot_lf1,bratrq_mot_lf2));
            
            bratrq_mot_lr1=bratrq_dem_lr*(v_act-v_thr1_b)/(v_thr2_b-v_thr1_b);
            bratrq_mot_lr2=9549*(pwr_chg_bat/4)/speed_act_lr;
            bratrq_mot_lr=min(trqlimL_dig_lr,min(bratrq_mot_lr1,bratrq_mot_lr2));
            
            bratrq_mot_rf1=bratrq_dem_rf*(v_act-v_thr1_b)/(v_thr2_b-v_thr1_b);
            bratrq_mot_rf2=9549*(pwr_chg_bat/4)/speed_act_rf;
            bratrq_mot_rf=min(trqlimL_dig_rf,min(bratrq_mot_rf1,bratrq_mot_rf2));
            
            bratrq_mot_rr1=bratrq_dem_rr*(v_act-v_thr1_b)/(v_thr2_b-v_thr1_b);
            bratrq_mot_rr2=9549*(pwr_chg_bat/4)/speed_act_rr;
            bratrq_mot_rr=min(trqlimL_dig_rr,min(bratrq_mot_rr1,bratrq_mot_rr2));
            
            brapre_out_l=((bratrq_dem_lf+bratrq_dem_lr)-(bratrq_mot_lf+bratrq_mot_lr))/150;
            brapre_out_r=((bratrq_dem_rf+bratrq_dem_rr)-(bratrq_mot_rf+bratrq_mot_rr))/150;
        else  %车速大于20，优先电制动,且进行ABS功能
            bratrq_mot_lf1=bratrq_dem_lf;
            bratrq_mot_lf2=9549*(pwr_chg_bat/4)/speed_act_lf;
            bratrq_mot_lf=min(trqlimL_dig_lf,min(bratrq_mot_lf1,bratrq_mot_lf2))+(bratrq_pid_lf-bratrq_dem_lf);
            
            bratrq_mot_rf1=bratrq_dem_rf;
            bratrq_mot_rf2=9549*(pwr_chg_bat/4)/speed_act_rf;
            bratrq_mot_rf=min(trqlimL_dig_rf,min(bratrq_mot_rf1,bratrq_mot_rf2))+(bratrq_pid_rf-bratrq_dem_rf);
            
            if (bratrq_pid_lr-bratrq_dem_lr)>(bratrq_pid_rr-bratrq_dem_rr)
                
                bratrq_mot_lr1=bratrq_dem_lr;
                bratrq_mot_lr2=9549*(pwr_chg_bat/4)/speed_act_lr;
                bratrq_mot_lr=min(trqlimL_dig_lr,min(bratrq_mot_lr1,bratrq_mot_lr2))+(bratrq_pid_rr-bratrq_dem_rr);
                
                
                
                bratrq_mot_rr1=bratrq_dem_rr;
                bratrq_mot_rr2=9549*(pwr_chg_bat/4)/speed_act_rr;
                bratrq_mot_rr=min(trqlimL_dig_rr,min(bratrq_mot_rr1,bratrq_mot_rr2))+(bratrq_pid_rr-bratrq_dem_rr);
                
                brapre_out_l=((bratrq_pid_lf+bratrq_dem_lr-(bratrq_pid_rr-bratrq_dem_rr))-(bratrq_mot_lf+bratrq_mot_lr))/150;
                brapre_out_r=((bratrq_pid_rf+bratrq_pid_rr)-(bratrq_mot_rf+bratrq_mot_rr))/150;
            else
                bratrq_mot_lr1=bratrq_dem_lr;
                bratrq_mot_lr2=9549*(pwr_chg_bat/4)/speed_act_lr;
                bratrq_mot_lr=min(trqlimL_dig_lr,min(bratrq_mot_lr1,bratrq_mot_lr2))+(bratrq_pid_lr-bratrq_dem_lr);
                
                
                
                bratrq_mot_rr1=bratrq_dem_rr;
                bratrq_mot_rr2=9549*(pwr_chg_bat/4)/speed_act_rr;
                bratrq_mot_rr=min(trqlimL_dig_rr,min(bratrq_mot_rr1,bratrq_mot_rr2))+(bratrq_pid_lr-bratrq_dem_lr);
                
                brapre_out_l=((bratrq_pid_lf+bratrq_pid_lr)-(bratrq_mot_lf+bratrq_mot_lr))/150;
                brapre_out_r=((bratrq_pid_rf+bratrq_dem_rr-(bratrq_pid_lr-bratrq_dem_lr))-(bratrq_mot_rf+bratrq_mot_rr))/150;
            end
        end
    end
    
    
    
end
end
